simulink subsystem "microcontroller"  (R2025a)
settings: Solver=VariableStepAuto  StartTime=0.0  StopTime=10.0  RelTol=1e-3
settings Model: Creator=Глеб  LastModifiedBy=Глеб

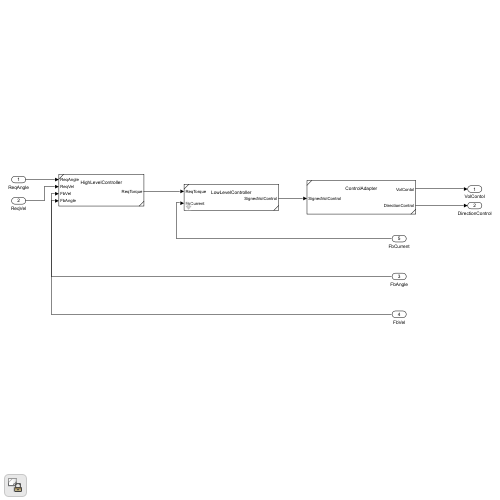
[thumbnail: Simulink's stored preview of the top-level diagram]
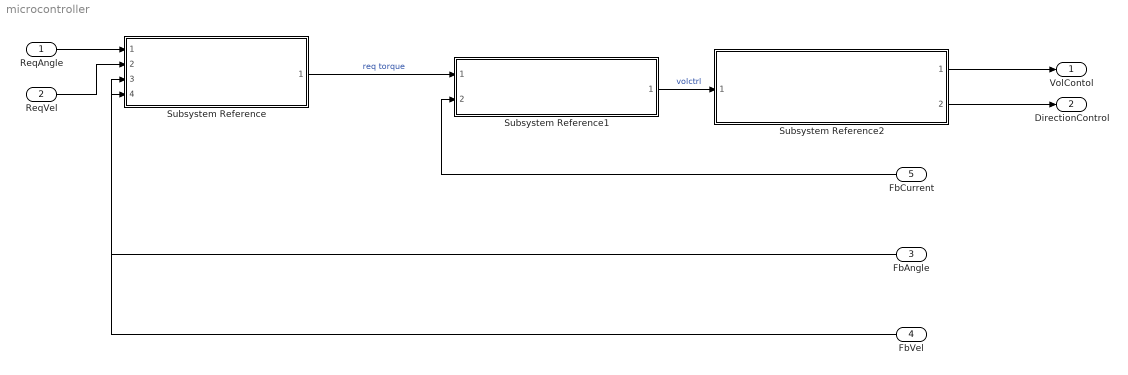
== system microcontroller ==
  ReqAngle : Inport
  ReqVel : Inport  Port=2
  FbAngle : Inport  Port=3
  FbVel : Inport  Port=4
  FbCurrent : Inport  Port=5
  Subsystem Reference : Subsystem  ReferencedSubsystem=HighLevelController
  Subsystem Reference1 : Subsystem  ReferencedSubsystem=LowLevelController  motor_km=16/1000
  Subsystem Reference2 : Subsystem  ReferencedSubsystem=ControlAdapter
  VolContol : Outport
  DirectionControl : Outport  Port=2
  wires:
  FbAngle/1 -> Subsystem Reference/4
  FbCurrent/1 -> Subsystem Reference1/2
  Subsystem Reference2/2 -> DirectionControl/1
  ReqVel/1 -> Subsystem Reference/2
  Subsystem Reference1/1 -> Subsystem Reference2/1  "volctrl"
  ReqAngle/1 -> Subsystem Reference/1
  Subsystem Reference2/1 -> VolContol/1
  FbVel/1 -> Subsystem Reference/3
  Subsystem Reference/1 -> Subsystem Reference1/1  "req torque"
